simulink model "control_model"  (R2015a)
settings: Solver=ode45  StartTime=0  StopTime=1000  FixedStep=0.01  RelTol=1e-3
settings Model: Creator=keysie  LastModifiedBy=keysie

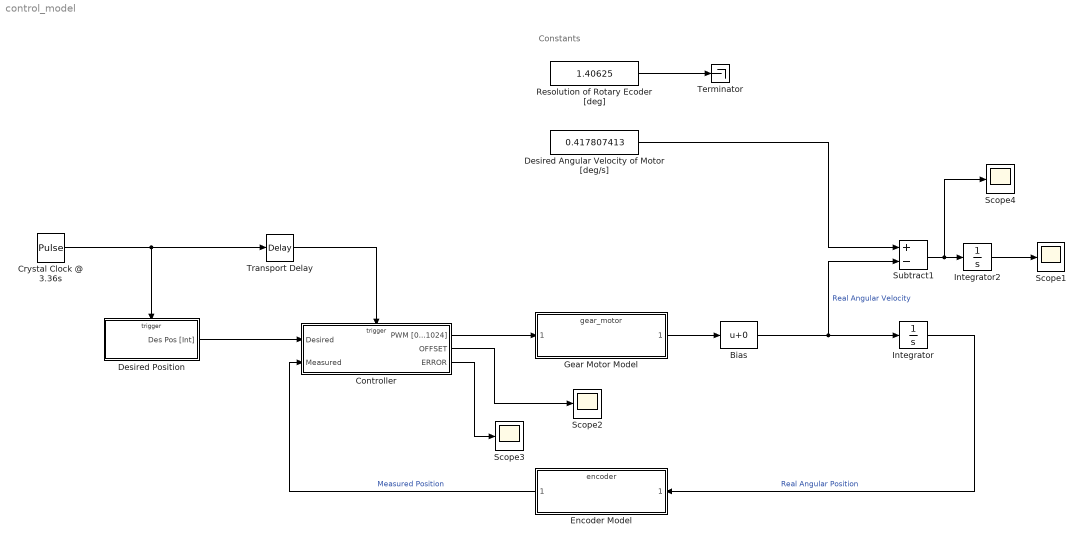
== system control_model ==
  note: Constants
  Bias : Bias
  Controller : Subsystem  TreatAsAtomicUnit=on
  Crystal Clock @ 3.36s : DiscretePulseGenerator  PulseType=Time based  Period=3.365785183  PulseWidth=5
  Desired Angular Velocity of Motor [deg/s] : Constant  Value=0.417807413
  Desired Position : Subsystem  TreatAsAtomicUnit=on
  Encoder Model : ModelReference  ModelNameDialog=encoder.slx  SimulationMode=Normal  ModelReferenceVersion=1.7  CopyOfModelName=encoder.slx  DefaultDataLogging=on
  Gear Motor Model : ModelReference  ModelNameDialog=gear_motor.slx  SimulationMode=Normal  ModelReferenceVersion=1.24  CopyOfModelName=gear_motor.slx  DefaultDataLogging=on
  Integrator : Integrator
  Integrator2 : Integrator
  Resolution of Rotary Ecoder [deg] : Constant  Value=1.40625
  Scope{1..4} (4 alike) : Scope
      Scope1 settings: TimeRange=1000
      Scope2 settings: TimeRange=100  SaveName=ScopeData2
      Scope3 settings: SaveName=ScopeData6
      Scope4 settings: TimeRange=1000
  Subtract1 : Sum  Inputs=+-
  Terminator : Terminator
  Transport Delay : TransportDelay  DelayTime=0.01
  wires:
  Gear Motor Model/1 -> Bias/1
  Integrator/1 -> Encoder Model/1  "Real Angular Position"
  Encoder Model/1 -> Controller/2(Measured)  "Measured Position"
  Crystal Clock @ 3.36s/1 -> Desired Position/Trigger, Transport Delay/1
  Desired Position/1(Des Pos [Int]) -> Controller/1(Desired)
  Controller/1(PWM [0...1024]) -> Gear Motor Model/1
  Controller/2(OFFSET) -> Scope2/1
  Subtract1/1 -> Scope4/1, Integrator2/1
  Integrator2/1 -> Scope1/1
  Controller/3(ERROR) -> Scope3/1
  Transport Delay/1 -> Controller/Trigger
  Desired Angular Velocity of Motor [deg/s]/1 -> Subtract1/1
  Resolution of Rotary Ecoder [deg]/1 -> Terminator/1
  Bias/1 -> Integrator/1, Subtract1/2  "Real Angular Velocity"

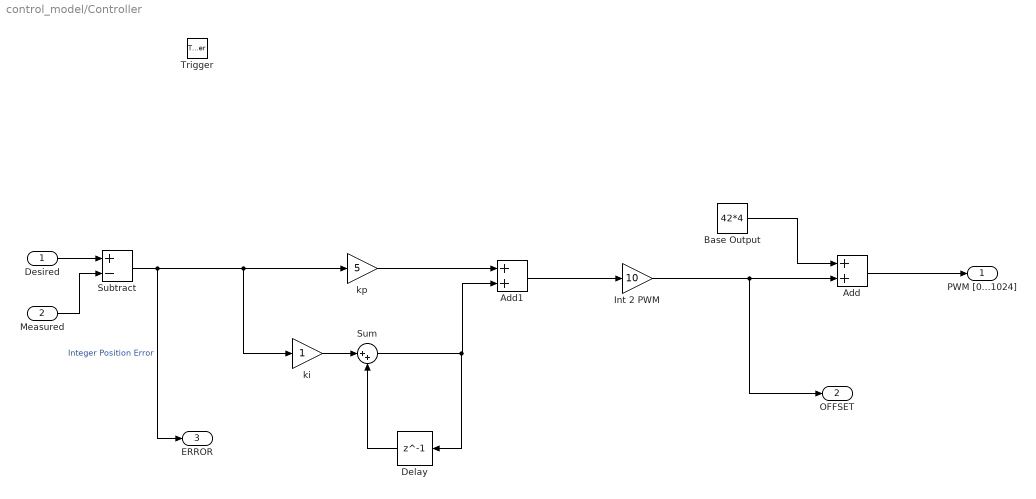
== system control_model/Controller ==
  Desired : Inport
  Measured : Inport  Port=2
  Trigger : TriggerPort
  Add : Sum
  Add1 : Sum
  Base Output : Constant  Value=42*4
  Delay : Delay  DelayLength=1
  Int 2 PWM : Gain  Gain=10
  Subtract : Sum  Inputs=+-
  Sum : Sum  Inputs=|++
  ki : Gain
  kp : Gain  Gain=5
  PWM [0...1024] : Outport  InitialOutput=[0]
  OFFSET : Outport  Port=2  InitialOutput=[0]
  ERROR : Outport  Port=3  InitialOutput=[0]
  wires:
  Base Output/1 -> Add/1
  Add/1 -> PWM [0...1024]/1
  Subtract/1 -> ERROR/1, ki/1, kp/1  "Integer Position Error"
  kp/1 -> Add1/1
  ki/1 -> Sum/1
  Add1/1 -> Int 2 PWM/1
  Int 2 PWM/1 -> OFFSET/1, Add/2
  Sum/1 -> Delay/1, Add1/2
  Delay/1 -> Sum/2
  Desired/1 -> Subtract/1
  Measured/1 -> Subtract/2

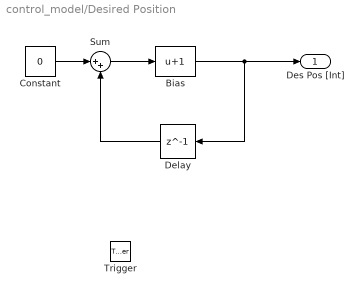
== system control_model/Desired Position ==
  Trigger : TriggerPort
  Bias : Bias  Bias=1
  Constant : Constant  Value=0
  Delay : Delay  DelayLength=1
  Sum : Sum  Inputs=|++
  Des Pos [Int] : Outport  InitialOutput=[0]
  wires:
  Bias/1 -> Delay/1, Des Pos [Int]/1
  Delay/1 -> Sum/2
  Constant/1 -> Sum/1
  Sum/1 -> Bias/1
